simulink model "DC_Motor_control_of_speed"  (R2016a)
settings: Solver=VariableStepAuto  StartTime=0.0  StopTime=40  RelTol=1e-3
libraries: powerlib x5, simulink x1
settings Model: Creator=AT Once  LastModifiedBy=AT Once

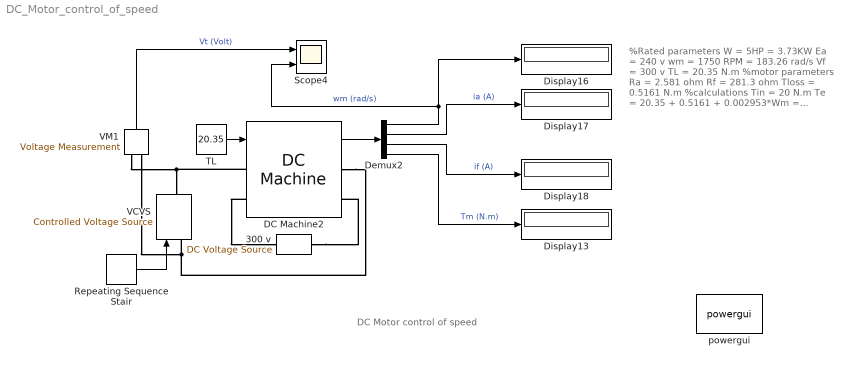
== system DC_Motor_control_of_speed ==
  note: DC Motor control of speed
  note: %Rated parameters
      | W = 5HP = 3.73KW
      | Ea = 240 v
      | wm = 1750 RPM = 183.26 rad/s
      | Vf = 300 v
      | TL = 20.35 N.m
      |
      | %motor parameters
      | Ra = 2.581 ohm
      | Rf = 281.3 ohm
      | Tloss = 0.5161 N.m
      |
      | %calculations
      | Tin = 20 N.m
      | Te = 20.35 + 0.5161 + 0.002953*Wm =
      | 21.407 N.m
  300 v : powerlib/Electrical Sources/DC Voltage Source  Amplitude=300  Measurements=None
  DC Machine2 : powerlib/Machines/DC Machine  PresetModel=01: 5HP 240V 1750RPM Field:300V  MechanicalLoad=Torque TL  FieldType=Wound  ShowDetailedParameters=on  MeasurementBus=off  RLa=[2.581 0.028]  RLf=[281.3 156]  Laf=0.9483  MachineConstant=Torque constant (N.m/A)  Ke=1.8  Kt=1.8  J=0.02215  Bm=0.002953  Tf=0.5161  w0=0  Ifinit=0  TsPowergui=0  TsBlock=-1
  Demux2 : Demux
  Display{13,16..18} (4 alike) : Display
  Repeating Sequence Stair : simulink/Sources/Repeating Sequence Stair  OutValues=[0 80 160 240].'  tsamp=10  OutMin=[]  OutMax=[]  OutDataTypeStr=double  OutputDataTypeScalingMode=double  OutDataType=fixdt(0,8)  ConRadixGroup=Best Precision: Vector-wise  OutScaling=2^-12
  Scope4 : Scope  NumInputPorts=2
  TL : Constant  Value=20.35
  VCVS : powerlib/Electrical Sources/Controlled Voltage Source  Initialize=on  Source_Type=AC  Amplitude=0  Phase=0  Frequency=0  Measurements=None
  VM1 : powerlib/Measurements/Voltage Measurement  PhasorSimulation=off  OutputType=Complex  PSBequivalent=0
  powergui : powerlib/powergui  Priority=1  SimulationMode=Discrete  SolverType=Tustin/Backward Euler (TBE)  SampleTime=50e-6  frequency=60  SPID=off  DisableSnubberDevices=off  DisableRonSwitches=off  DisableVfSwitches=off  SwTol=0  DisplayEquations=off  Interpol=off  ExternalGateDelay=off  methode=off  Ts=10  FunctionMessages=off  echomessages=off  HookPort=off  EnableUseOfTLC=off  x0status=blocks  frequencyindice=0  Pbase=100e6  ErrMax=1e-4  Iterations=50  UnitsV=kV  UnitsW=MW  buscounter=0  RestoreLinks=warning  ResistiveCurrentMeasurement=off  Frange=[0:2:500]  Ylog=off  Xlog=on  ShowGrid=off  save=off  variable=ZData  structure=0  ZoomFFT=off  StartTime=0.0  cycles=1  DisplayStyle=1  fundamental=60  FreqAxis=off  MaxFrequency=1000  frequencyindicesteady=1  RmsSteady=1  display=off
  wires:
  DC Machine2/1 -> Demux2/1
  Demux2/1 -> Scope4/2, Display16/1  "wm (rad/s)"
  Demux2/2 -> Display17/1  "ia (A)"
  Demux2/3 -> Display18/1  "if (A)"
  Demux2/4 -> Display13/1  "Tm (N.m)"
  TL/1 -> DC Machine2/1
  VM1/1 -> Scope4/1  "Vt (Volt)"
  Repeating Sequence Stair/1 -> VCVS/1
  connections:
  DC Machine2/LConn1 -- VM1/LConn1 -- VCVS/RConn1
  DC Machine2/RConn1 -- VM1/LConn2 -- VCVS/LConn1
  300 v/LConn1 -- DC Machine2/RConn2
  DC Machine2/LConn2 -- 300 v/RConn1
